simulink model "errorcoding_example"  (R2018b)
settings: Solver=ode45  StartTime=0.0  StopTime=1  RelTol=1e-3  EnableMultiTasking=on
undefined symbols (not defined in the file): gfprimfd
libraries: commblkcod2 x2, commdigbbndfm2 x2, commchan3 x1, commsink2 x1, commrandsrc2 x1
settings Model: Creator=Ammar  LastModifiedBy=ahmedmohamud
settings DataIOCC: LimitDataPoints=on  SaveFormat=Array  SignalLoggingSaveFormat=ModelDataLogs
settings OptimizationCC: ExpressionDepthLimit=2147483647  LifeSpan=inf
settings DebuggingCC: UnderspecifiedInitializationDetection=Classic  MergeDetectMultiDrivingBlocksExec=none  SolverPrmCheckMsg=warning  FcnCallInpInsideContextMsg=warning  StateNameClashWarn=warning  SFUnexpectedBacktrackingDiag=warning  SFNoUnconditionalDefaultTransitionDiag=warning  SFExecutionAtInitializationDiag=none
settings HardwareCC: ProdBitPerPointer=32  ProdBitPerSizeT=32  ProdBitPerPtrDiffT=32  ProdLargestAtomicFloat=None  ProdIntDivRoundTo=Undefined  ProdEndianess=Unspecified  ProdWordSize=32  ProdHWDeviceType=32-bit Generic
settings ModelReferenceCC: PropagateSignalLabelsOutOfModel=off
settings SFSimCC: SimUseLocalCustomCode=off
settings RTWCC: RTWUseLocalCustomCode=off
settings CodeAppCC: StateflowObjectComments=on
settings GRTTargetCC: TargetLangStandard=C89/C90 (ANSI)  GeneratePreprocessorConditionals=Disable all  CombineOutputUpdateFcns=off  GRTInterface=on
settings ConfigComp: CovMetricSettings=dw  CovHtmlReporting=on  CovSaveCumulativeToWorkspaceVar=on  CovSaveSingleToWorkspaceVar=on  CovExternalEMLEnable=off  CovSFcnEnable=off

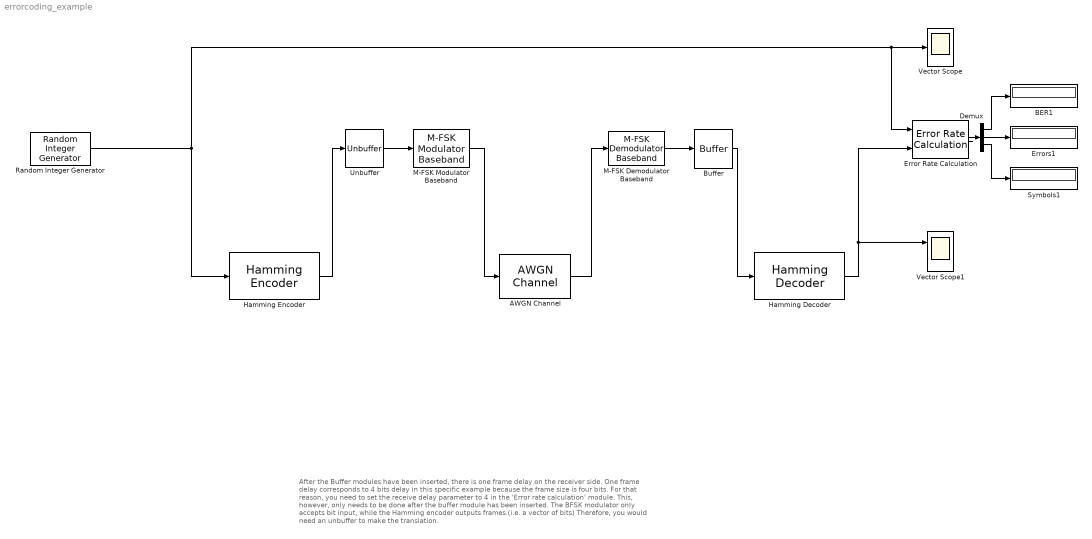
== system errorcoding_example ==
  note: After the Buffer modules have been inserted, there is one frame delay on the receiver side. One frame delay corresponds to 4 bits delay in this specific example
      | because the frame size is four bits.
      | For that reason, you need to set the receive delay parameter to 4 in the 'Error rate calculation' module. This, however, only needs to be done after the buffer module
      | has been inserted.
      | The BFSK modulator only accepts bit input, while the Hamming encoder outputs frames.(i.e. a vector of bits) Therefore, you would need an unbuffer to make the translation.
  AWGN Channel : commchan3/AWGN Channel  InputProcessing=Columns as channels (frame based)  seed=67  noiseMode="Signal to noise ratio  (Eb/No)"  EbNodB=10  EsNodB=6  SNRdB=10  bitsPerSym=1  Ps=1  Tsym=1/10000  variance=1
      settings: SourceProductName=Communications Toolbox
  BER1 : Display
  Buffer : Buffer  N=7
  Demux : Demux  Outputs=3
  Error Rate Calculation : commsink2/Error Rate Calculation  N=4  st_delay=0  cp_mode=Entire frame  subframe=[]  PMode=Port  WsName=ErrorVec  RsMode2=off  stop=off  numErr=100  maxBits=1e6
      settings: SourceProductName=Communications Toolbox
  Errors1 : Display
  Hamming Decoder : commblkcod2/Hamming Decoder  n=7  k=gfprimfd(3,'min')
      settings: SourceProductName=Communications Toolbox  SourceProductBaseCode=CM
  Hamming Encoder : commblkcod2/Hamming Encoder  n=7  k=gfprimfd(3,'min')
      settings: SourceProductName=Communications Toolbox  SourceProductBaseCode=CM
  M-FSK Demodulator Baseband : commdigbbndfm2/M-FSK Demodulator Baseband  M=2  OutType=Bit  Dec=Gray  freqSep=60  numSamp=10  RateOptions=Enforce single-rate processing  outDataType=double
      settings: SourceProductName=Communications Toolbox  SourceProductBaseCode=CM
  M-FSK Modulator Baseband : commdigbbndfm2/M-FSK Modulator Baseband  M=2  InType=Bit  Enc=Binary  freqSep=60  phaseType=Continuous  numSamp=10  RateOptions=Enforce single-rate processing  outDataType=double
      settings: SourceProductName=Communications Toolbox
  Random Integer Generator : commrandsrc2/Random Integer Generator  mul=2  seed=37  Ts=1/10000  frameBased=on  sampPerFrame=4  orient=off  outDataType=double
  Symbols1 : Display
  Unbuffer : Unbuffer
  Vector Scope : Scope
  Vector Scope1 : Scope  NumInputPorts=2
  wires:
  Random Integer Generator/1 -> Hamming Encoder/1, Error Rate Calculation/1, Vector Scope/1
  Demux/1 -> BER1/1
  Demux/2 -> Errors1/1
  Demux/3 -> Symbols1/1
  Error Rate Calculation/1 -> Demux/1
  Hamming Decoder/1 -> Error Rate Calculation/2, Vector Scope1/1
  Hamming Encoder/1 -> Unbuffer/1
  M-FSK Modulator Baseband/1 -> AWGN Channel/1
  Unbuffer/1 -> M-FSK Modulator Baseband/1
  Buffer/1 -> Hamming Decoder/1
  AWGN Channel/1 -> M-FSK Demodulator Baseband/1
  M-FSK Demodulator Baseband/1 -> Buffer/1
